simulink model "conversion_example"  (R2017b)
settings: Solver=VariableStepAuto  StartTime=0.0  StopTime=10.0  RelTol=1e-3
undefined symbols (not defined in the file): Phase, Single, Split, typhoonPatterns, VSI
libraries: typhoonHILlib x5, powerlib x2
settings Model: Creator=Marcos  LastModifiedBy=Marcos

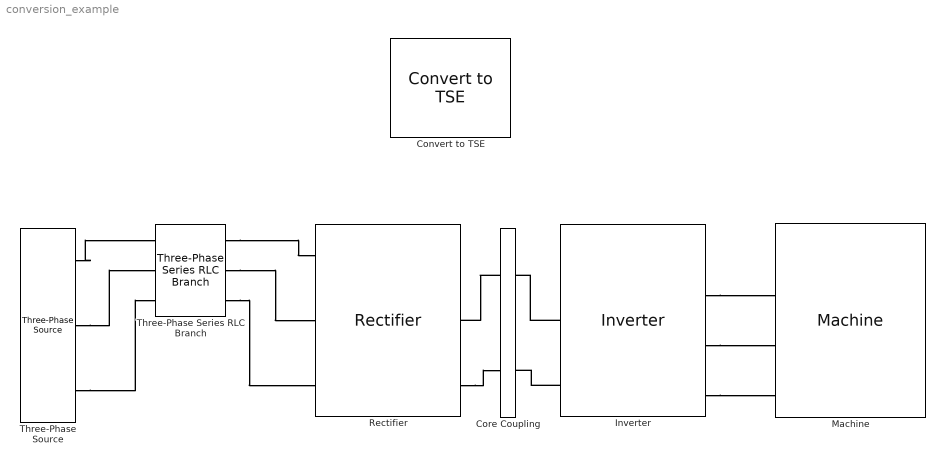
== system conversion_example ==
  Convert to TSE : typhoonHILlib/Convert to TSE  versions=C:\Program Files\Typhoon HIL Control Center 2020.1 alpha25  device=HIL402  compile=on  toggle_init=on
      settings: SourceProductName=Typhoon HIL
  Core Coupling : typhoonHILlib/Core Coupling  CouplingPhases=Single-Phase  IsTLM=off  snb_type_i=None  R1=100000  C1=1e-6  fixed_snb_i=off  snb_type_v=None  R2=0.1  L1=0.1  fixed_snb_v=off  CouplingType=Inductive  coup_cap=1e-3  coup_ind=1e-3  toggle_init=on  model_loaded=off  old_pat=typhoonPatterns/SP CC  old_size=15,189
      settings: SourceProductName=Typhoon HIL
  Inverter : typhoonHILlib/Inverter  InvType=VSI  ThreePhase=on  sa1_logic=Active-high  sa2_logic=Active-high  sa3_logic=Active-high  sa4_logic=Active-high  sa5_logic=Active-high  sa6_logic=Active-high  sb1_logic=Active-high  sb2_logic=Active-high  sb3_logic=Active-high  sb4_logic=Active-high  sb5_logic=Active-high  sb6_logic=Active-high  sc1_logic=Active-high  sc2_logic=Active-high  sc3_logic=Active-high  sc4_logic=Active-high  sc5_logic=Active-high  sc6_logic=Active-high  di_sa1=1  di_sa2=7  di_sa3=2  di_sa4=8  di_sa5=3  di_sa6=9  di_sb1=7  di_sb2=8  di_sb3=9  di_sb4=10  di_sb5=11  di_sb6=12  di_sc1=13  di_sc2=14  di_sc3=15  di_sc4=16  di_sc5=17  di_sc6=18  v_sa1=on  v_sa2=off  v_sa3=off  v_sa4=off  v_sa5=off  v_sa6=off  v_sb1=off  v_sb2=off  v_sb3=off  v_sb4=off  v_sb5=off  v_sb6=off  v_sc1=off  v_sc2=off  v_sc3=off  v_sc4=off  v_sc5=off  v_sc6=off  i_sa1=off  i_sa2=off  i_sa3=off  i_sa4=off  i_sa5=off  i_sa6=off  i_sb1=off  i_sb2=off  i_sb3=off  i_sb4=off  i_sb5=off  i_sb6=off  i_sc1=off  i_sc2=off  i_sc3=off  i_sc4=off  i_sc5=off  i_sc6=off  c_clamp=1e-6  v0_clamp=0  r_clamp=1e-4  r_on=0.001  v_f=0  r_s=1e5  c_s=inf  toggle_init=on  toggle_draw=on  model_loaded=off  old_pat=typhoonPatterns/VSI (3-Phase)  old_size=145,192
      settings: SourceProductName=Typhoon HIL
  Machine : typhoonHILlib/Machine  MachineType=Induction Machine  RotorType_PMSM=Salient Pole  RotorType_Ind=Squirrel Cage  sp_ind=off  vbr=off  Rsnb_stator=20e3  Rsnb_rotor=20e3  theta_ab=-pi/2  Rs_pmsm=2.35  Ld_pmsm=7e-3  Lq_pmsm=3e-3  Lms_pmsm=1e-3  psi_pm_pmsm=0.30204  Rs_ind=9.173  Rr_ind=6.422  Rr1_ind=11.202  Rr2_ind=11.202  Rrc_ind=0  Lls_ind=0.01889  Llr_ind=0.01889  Llr1_ind=0.0194  Llr2_ind=0.0194  Lm_ind=0.3203  Lmr_ind=0  Ra_DC=2.581  Rf_DC=281.3  La_DC=0.028  Lf_DC=156.0  Laf_DC=0.9483  sp_start_type=Split-Phase  f_sp_ind=50  rsm_sp_ind=2.02  llsm_sp_ind=7.4e-3  rsa_sp_ind=7.14  llsa_sp_ind=8.5e-3  lmm_sp_ind=0.1772  rrm_sp_ind=4.12  llrm_sp_ind=5.6e-3  nanm_sp_ind=1.18  rst_sp_ind=2  cst_sp_ind=254.7e-6  rrun_sp_ind=18  crun_sp_ind=21.1e-6  pms=2  Jm=0.0023  fc=0  w_disc=75  stardelta=Star  uc_mech_angle=off  loadtype=Torque  loadsource=SCADA / external  load_ai=1  load_offset=0  load_gain=1  ppr=1000  resolver_pp=1  resolver_source=Internal  resolver_freq=5e3  resolver_ai=1  resolver_offset=0  resolver_gain=1  toggle_init=on  toggle_draw=off  model_loaded=off  old_pat=typhoonPatterns/Induction Machine  old_size=150,194
      settings: SourceProductName=Typhoon HIL
  Rectifier : typhoonHILlib/Rectifier  RecType=Diode  ThreePhase=on  sa_top_logic=Active-high  sa_bot_logic=Active-high  sb_top_logic=Active-high  sb_bot_logic=Active-high  sc_top_logic=Active-high  sc_bot_logic=Active-high  di_sa_top=1  di_sa_bot=2  di_sb_top=3  di_sb_bot=4  di_sc_top=5  di_sc_bot=6  v_sa_top=off  i_sa_top=on  v_sa_bot=off  i_sa_bot=off  v_sb_top=off  i_sb_top=off  v_sb_bot=off  i_sb_bot=off  v_sc_top=off  i_sc_top=off  v_sc_bot=off  i_sc_bot=off  r_on=0.001  v_f=0  r_s=1e5  c_s=inf  toggle_init=on  toggle_draw=on  model_loaded=off  old_pat=typhoonPatterns/Diode Rectifier (3-Phase)  old_size=145,192
      settings: SourceProductName=Typhoon HIL
  Three-Phase Series RLC Branch : powerlib/Elements/Three-Phase Series RLC Branch  LConnTagsString=A|B|C  RConnTagsString=A|B|C  BranchType=RLC  Resistance=1  Inductance=1e-3  Capacitance=1e-6  Measurements=None
  Three-Phase Source : powerlib/Electrical Sources/Three-Phase Source  InternalConnection=Yg  VoltagePhases=off  Voltage=230  PhaseAngle=0  Voltage_phases=[25e3 25e3 25e3]/sqrt(3)  PhaseAngles_phases=[0 -120 +120]  Frequency=60  NonIdealSource=off  SpecifyImpedance=off  Resistance=0.8929  Inductance=16.58e-3  ShortCircuitLevel=100e6  BaseVoltage=25e3  XRratio=7  BusType=swing  Pref=10e3  Qref=0  Prefabc=[10e3, 10e3, 10e3]  Qrefabc=[0, 0, 0]  Qmin=-inf  Qmax=inf
  connections:
  Inverter/LConn1 -- Core Coupling/RConn1
  Inverter/LConn2 -- Core Coupling/RConn2
  Three-Phase Series RLC Branch/RConn3 -- Rectifier/LConn3
  Three-Phase Series RLC Branch/RConn2 -- Rectifier/LConn2
  Three-Phase Source/RConn1 -- Three-Phase Series RLC Branch/LConn1
  Three-Phase Source/RConn2 -- Three-Phase Series RLC Branch/LConn2
  Three-Phase Source/RConn3 -- Three-Phase Series RLC Branch/LConn3
  Three-Phase Series RLC Branch/RConn1 -- Rectifier/LConn1
  Inverter/RConn3 -- Machine/LConn3
  Inverter/RConn2 -- Machine/LConn2
  Inverter/RConn1 -- Machine/LConn1
  Rectifier/RConn2 -- Core Coupling/LConn2
  Core Coupling/LConn1 -- Rectifier/RConn1
